simulink model "Project_simulink"  (R2018b)
settings: Solver=FixedStepAuto  StartTime=0.0  StopTime=inf  RelTol=1e-3  EnableMultiTasking=on
libraries: arduinolib x9
settings Model: ExtModeTrigDuration=2  Creator=FatmaGomaa  LastModifiedBy=FatmaGomaa
settings OptimizationCC: EnhancedBackFolding=on  PassReuseOutputArgsAs=Individual arguments  MaxStackSize=64  OptimizeBlockOrder=speed  DifferentSizesBufferReuse=on  OptimizationCustomize=off
settings DebuggingCC: ParameterTunabilityLossMsg=error
settings HardwareCC: ProdBitPerInt=16  ProdBitPerPointer=16  ProdBitPerSizeT=16  ProdBitPerPtrDiffT=16  ProdLargestAtomicFloat=None  ProdWordSize=8  ProdHWDeviceType=Atmel->AVR
settings SFSimCC: MATLABDynamicMemAlloc=off
settings RTWCC: SystemTargetFile=ert.tlc  HardwareBoard=Arduino Uno  TemplateMakefile=ert_default_tmf  GenerateReport=on  Toolchain=Arduino AVR  BuildConfiguration=Faster Runs  IncludeHyperlinkInReport=on  LaunchReport=on  GenerateTraceInfo=on  GenerateTraceReport=on  GenerateTraceReportSl=on  GenerateTraceReportSf=on  GenerateTraceReportEml=on
settings CodeAppCC: ForceParamTrailComments=on  IgnoreCustomStorageClasses=off  OperatorAnnotations=on  SimulinkDataObjDesc=on  SFDataObjDesc=on  InsertBlockDesc=on
settings ERTTargetCC: SupportContinuousTime=on  SupportVariableSizeSignals=on

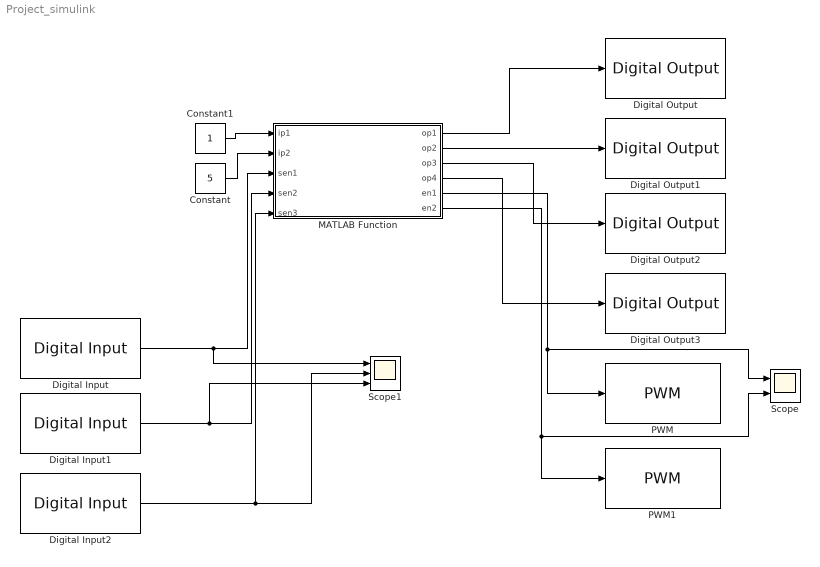
== system Project_simulink ==
  Constant : Constant  Value=5
  Constant1 : Constant
  Digital Input : arduinolib/Digital Input  pinNumber=3  sampleTime=1  blockPlatform=arduino
      settings: SourceProductName=Simulink Support Package for Arduino Hardware
  Digital Input1 : arduinolib/Digital Input  pinNumber=4  sampleTime=1  blockPlatform=arduino
      settings: SourceProductName=Simulink Support Package for Arduino Hardware
  Digital Input2 : arduinolib/Digital Input  pinNumber=5  sampleTime=1  blockPlatform=arduino
      settings: SourceProductName=Simulink Support Package for Arduino Hardware
  Digital Output : arduinolib/Digital Output  pinNumber=12  blockPlatform=arduino
  Digital Output1 : arduinolib/Digital Output  pinNumber=13  blockPlatform=arduino
  Digital Output2 : arduinolib/Digital Output  pinNumber=8  blockPlatform=arduino
  Digital Output3 : arduinolib/Digital Output  pinNumber=9  blockPlatform=arduino
  MATLAB Function : MATLAB Function  TreatAsAtomicUnit=on
  PWM : arduinolib/PWM  pinNumber=10  EnableInputFrequency=off  InitialFrequency=2000  InitialDutyCycle=0  NotificationType=None  blockPlatform=arduino
  PWM1 : arduinolib/PWM  pinNumber=11  EnableInputFrequency=off  InitialFrequency=2000  InitialDutyCycle=0  NotificationType=None  blockPlatform=arduino
  Scope : Scope  NumInputPorts=2
  Scope1 : Scope  NumInputPorts=3
  wires:
  MATLAB Function/1(op1) -> Digital Output/1
  MATLAB Function/2(op2) -> Digital Output1/1
  MATLAB Function/3(op3) -> Digital Output2/1
  MATLAB Function/4(op4) -> Digital Output3/1
  MATLAB Function/5(en1) -> PWM/1, Scope/1
  MATLAB Function/6(en2) -> PWM1/1, Scope/2
  Constant1/1 -> MATLAB Function/1(ip1)
  Constant/1 -> MATLAB Function/2(ip2)
  Digital Input/1 -> Scope1/1, MATLAB Function/3(sen1)
  Digital Input1/1 -> Scope1/3, MATLAB Function/4(sen2)
  Digital Input2/1 -> Scope1/2, MATLAB Function/5(sen3)

== matlab function Project_simulink/MATLAB Function ==
  data: ip1 input; op1 output; op2 output; op3 output; op4 output; ip2 input; en1 output; en2 output; sen1 input; sen2 input; sen3 input
function [op1,op2,op3,op4,en1,en2] = fcn(ip1,ip2, sen1, sen2, sen3)
        %Manual, Forward Mode
        if (ip1 == 1 && ip2 == 1)
         op1 = 0;
         op2 = 1;
         op3 = 1;
         op4 = 0;
         en1 = 100;
         en2 = 100;
        %Manual, Backward Mode
        elseif (ip1 == 1 && ip2 == 2)
         op1 = 1;
         op2 = 0;
         op3 = 0;
         op4 = 1; 
         en1=100;
         en2=100;
        %Manual, Left Mode
        elseif (ip1 == 1 && ip2 == 3)
         op1 = 0;
         op2 = 1;
         op3 = 1;
         op4 = 0;
         en1=60;
         en2=100;
         %Manual, Right Mode
        elseif (ip1 == 1 && ip2 == 4)
         op1 = 0;
         op2 = 1;
         op3 = 1;
         op4 = 0;
         en1=100;
         en2=60;
        else
         op1 = 0;
         op2 = 0;
         op3 = 0;
         op4 = 0;
         en1 = 100;
         en2 = 100;
        end
         %LineFollower Mode
        if (ip1==2 )
            if (sen1 ==0 && sen2 == 1 && sen3 == 1)
         op1 = 0;
         op2 = 1;
         op3 = 1;
         op4 = 0;
         en1 = 100;
         en2 = 60;
            elseif (sen1 ==0 && sen2 == 0 && sen3 == 0)
         op1 = 0;
         op2 = 1;
         op3 = 1;
         op4 = 0;
         en1 = 100;
         en2 = 100;   
            elseif (sen1 ==1 && sen2 == 1 && sen3 == 0)
         op1 = 0;
         op2 = 1;
         op3 = 1;
         op4 = 0;
         en1 = 60;
         en2 = 100; 
            else 
                             op1 = 0;
         op2 = 0;
         op3 = 0;
         op4 = 0;
         en1 = 60;
         en2 = 100;               
            end
        end
end
